simulink model "VSDsimul"  (R2020a)
settings: Solver=ode45  StartTime=0.0  StopTime=100.0  MaxStep=2.0  RelTol=1e-3
values from neighbouring files (symbols this model uses):
  A = eval(a)    [VSDproject.m]
  B = eval(b)    [VSDproject.m]
  K = lqr(A,B,Q,R)    [VSDproject.m]
undefined symbols (not defined in the file or in its folder): C, D, sk
settings Model: Creator=Federico  LastModifiedBy=Federico

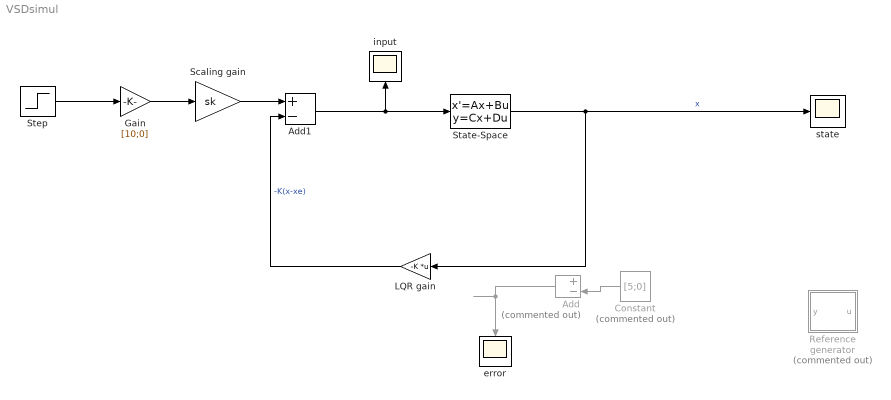
== system VSDsimul ==
  Add : Sum  Commented=on  Inputs=+-
  Add1 : Sum  Inputs=+-
  Constant : Constant  Commented=on  Value=[5;0]
  Gain : Gain  Gain=[10;0]
  LQR gain : Gain  Gain=-K  Multiplication=Matrix(K*u)
  Reference generator : MATLAB Function  Commented=on  TreatAsAtomicUnit=on
  Scaling gain : Gain  Gain=sk
  State-Space : StateSpace  A=A  B=B  C=C  D=D  InitialCondition=[100 ; 0]
  Step : Step  SampleTime=0
  error : Scope
  input : Scope
  state : Scope
  wires:
  State-Space/1 -> LQR gain/1, state/1  "x"
  Add/1 -> error/1
  Constant/1 -> Add/2
  Step/1 -> Gain/1
  Gain/1 -> Scaling gain/1
  Scaling gain/1 -> Add1/1
  LQR gain/1 -> Add1/2  "-K(x-xe)"
  Add1/1 -> State-Space/1, input/1

== matlab function VSDsimul/Reference generator ==
  data: u input; y output
function y = fcn(u)
y=u;
y(1)=5;
y(2)=0;
